simulink model "OberverForPMSM"  (R2018b)
settings: Solver=FixedStepAuto  StartTime=0.0  StopTime=inf  FixedStep=Ts  MaxStep=Ts  RelTol=1e-3  EnableMultiTasking=on
PreLoadFcn:
  | Ts=1e-6;
  | deci=20;
InitFcn:
  | Ts=5e-6;
  | deci=20;
undefined symbols (not defined in the file or in its folder): DiscIntNeverNeededParam, level
libraries: powerlib_extras x37, powerlib x18, powerlib_meascontrol x8, simulink x5, simulink_extras x4
(part 2 of 2)

== system OberverForPMSM/PMSG Wind Turbine/Control/Speed Control ==
  note: Speed Regulator
      | (Torque control)
  wr : Inport
  Enable : EnablePort
  0-inf1 : Saturate  UpperLimit=1.2  LowerLimit=0.7
  Divide2 : Product  Inputs=*/  SampleTime=Ts
  Gain1 : Gain  Gain=1/1.1^3  SampleTime=Ts
  Gain2 : Gain  Gain=-1  SampleTime=Ts
  Pmax : Constant
  Saturation1 : Saturate  UpperLimit=1  LowerLimit=0
  Saturation2 : Saturate  UpperLimit=1.5  LowerLimit=0
  Switch1 : Switch  Threshold=1.1
  Tracking Curve1 : Fcn  Expr=u(1)^3
  Tem_cmd : Outport
  wires:
  wr/1 -> 0-inf1/1, Divide2/2
  Pmax/1 -> Switch1/1
  0-inf1/1 -> Switch1/2, Tracking Curve1/1
  Switch1/1 -> Saturation1/1
  Divide2/1 -> Saturation2/1
  Saturation1/1 -> Divide2/1
  Tracking Curve1/1 -> Gain1/1
  Gain1/1 -> Switch1/3
  Saturation2/1 -> Gain2/1
  Gain2/1 -> Tem_cmd/1

== system OberverForPMSM/PMSG Wind Turbine/SMO_my/LL_To_Ph ==
  LL : Inport
  Selector : Selector  InputPortWidth=3  IndexOptions=Index vector (dialog)  Indices=[3 1 2]  OutputSizes=1
  Sum7 : Sum  Inputs=|+-
  constant : Gain  Gain=1/3
  Ph : Outport
  wires:
  LL/1 -> Sum7/1, Selector/1
  Selector/1 -> Sum7/2
  constant/1 -> Ph/1
  Sum7/1 -> constant/1

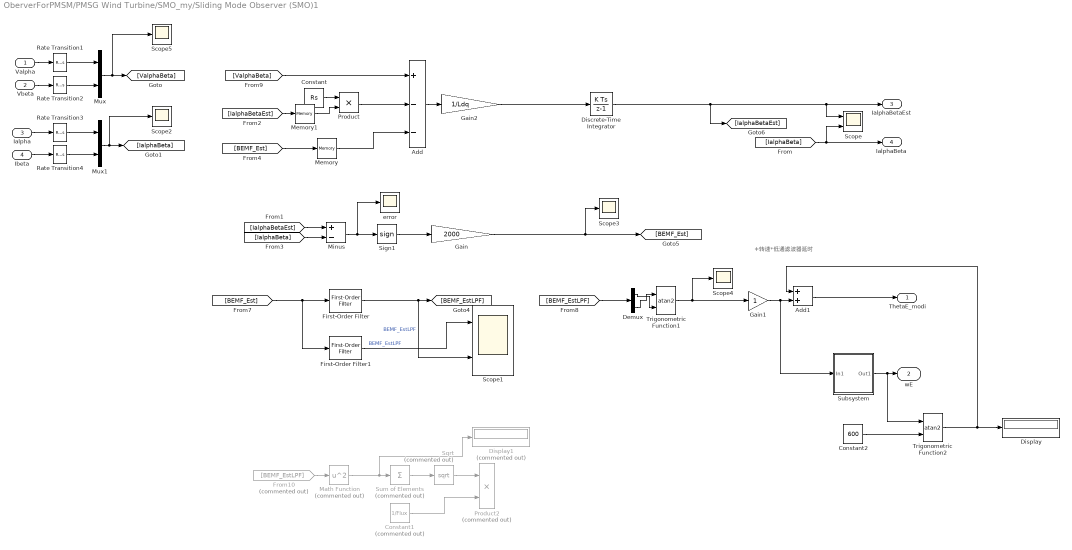
== system OberverForPMSM/PMSG Wind Turbine/SMO_my/Sliding Mode Observer (SMO)1 ==
  note: +转速*低通滤波器延时
  Valpha : Inport
  Vbeta : Inport  Port=2
  Ialpha : Inport  Port=3
  Ibeta : Inport  Port=4
  Add : Sum  Inputs=+--
  Add1 : Sum
  Constant : Constant  Value=Rs
  Constant1 : Constant  Commented=on  Value=1/Flux
  Constant2 : Constant  Value=600
  Demux : Demux  Outputs=2
  Discrete-Time Integrator : DiscreteIntegrator  SampleTime=-1  ICPrevOutput=DiscIntNeverNeededParam  ICPrevScaledInput=DiscIntNeverNeededParam
  Display : Display
  Display1 : Display  Commented=on
  First-Order Filter : powerlib_meascontrol/Filters/First-Order Filter  FilterType=Lowpass  Tc=1/600  Ts=Tctl  Initialize=on  Vac_Init=[0, 0, 60]  Vdc_Init=0  PlotResponse=off  FreqRange="[0,  200,  1]"
      settings: SourceProductName=Simscape Power Systems
  First-Order Filter1 : powerlib_meascontrol/Filters/First-Order Filter  FilterType=Lowpass  Tc=1/5000  Ts=Tctl  Initialize=on  Vac_Init=[0, 0, 60]  Vdc_Init=0  PlotResponse=off  FreqRange="[0,  200,  1]"
      settings: SourceProductName=Simscape Power Systems
  From10 : From  Commented=on  GotoTag=BEMF_EstLPF
  Gain : Gain  Gain=2000
  Gain1 : Gain
  Gain2 : Gain  Gain=1/Ldq
  Math Function : Math  Commented=on  Operator=square  SaturateOnIntegerOverflow=on
  Memory : Memory  InheritSampleTime=on
  Memory1 : Memory  InheritSampleTime=on
  Minus : Sum  Inputs=+-
  Mux : Mux  Inputs=2
  Mux1 : Mux  Inputs=2
  Product : Product
  Product2 : Product  Commented=on
  Rate Transition{1..4} (4 alike) : RateTransition  OutPortSampleTime=Tctl
  Scope : Scope  NumInputPorts=2
  Scope1 : Scope  NumInputPorts=2
  Scope{2..5} (4 alike) : Scope
  Sign1 : Signum
  Sqrt : Sqrt  Commented=on  SaturateOnIntegerOverflow=on
  Subsystem : Subsystem
  Sum of Elements : Sum  Commented=on  Inputs=+
  Trigonometric Function1 : Trigonometry  Operator=atan2  ApproximationMethod=CORDIC
  Trigonometric Function2 : Trigonometry  Operator=atan2  ApproximationMethod=CORDIC
  error : Scope
  ThetaE_modi : Outport
  wE : Outport  Port=2
  IalphaBetaEst : Outport  Port=3
  IalphaBeta : Outport  Port=4
  wires:
  Ibeta/1 -> Rate Transition4/1
  Ialpha/1 -> Rate Transition3/1
  Vbeta/1 -> Rate Transition2/1
  Valpha/1 -> Rate Transition1/1
  Mux/1 -> Scope5/1, [ValphaBeta]
  Mux1/1 -> Scope2/1, [IalphaBeta]
  [IalphaBetaEst] -> Minus/1
  [IalphaBeta] -> Minus/2
  [ValphaBeta] -> Add/1
  Constant/1 -> Product/1
  [IalphaBetaEst] -> Memory1/1
  Product/1 -> Add/2
  [BEMF_Est] -> Memory/1
  Add/1 -> Gain2/1
  Memory1/1 -> Product/2
  Gain2/1 -> Discrete-Time Integrator/1
  [IalphaBeta] -> Scope/2, IalphaBeta/1
  Minus/1 -> error/1, Sign1/1
  Memory/1 -> Add/3
  Sign1/1 -> Gain/1
  Gain/1 -> Scope3/1, [BEMF_Est]
  Trigonometric Function1/1 -> Scope4/1, Gain1/1
  Sum of Elements/1 -> Sqrt/1
  Math Function/1 -> Display1/1, Sum of Elements/1
  Sqrt/1 -> Product2/1
  Constant1/1 -> Product2/2
  From10/1 -> Math Function/1
  [BEMF_EstLPF] -> Demux/1
  Rate Transition1/1 -> Mux/1
  Rate Transition2/1 -> Mux/2
  Rate Transition3/1 -> Mux1/1
  Rate Transition4/1 -> Mux1/2
  [BEMF_Est] -> First-Order Filter1/1, First-Order Filter/1
  Discrete-Time Integrator/1 -> [IalphaBetaEst], Scope/1, IalphaBetaEst/1
  First-Order Filter/1 -> Scope1/2, [BEMF_EstLPF]  "BEMF_EstLPF"
  First-Order Filter1/1 -> Scope1/1  "BEMF_EstLPF"
  Subsystem/1(Out1) -> Trigonometric Function2/1, wE/1
  Demux/1 -> Trigonometric Function1/2
  Demux/2 -> Trigonometric Function1/1
  Gain1/1 -> Subsystem/1(In1), Add1/2
  Add1/1 -> ThetaE_modi/1
  Trigonometric Function2/1 -> Add1/1, Display/1
  Constant2/1 -> Trigonometric Function2/2

== system OberverForPMSM/PMSG Wind Turbine/SMO_my/mod 2 ==
  In1 : Inport
  Constant : Constant  Value=2*pi
  Math Function : Math  Operator=mod  SaturateOnIntegerOverflow=on
  Out1 : Outport
  wires:
  In1/1 -> Math Function/1
  Constant/1 -> Math Function/2
  Math Function/1 -> Out1/1

== system OberverForPMSM/PMSG Wind Turbine/SMO_my/mod 3 ==
  In1 : Inport
  Constant : Constant  Value=2*pi
  Math Function : Math  Operator=mod  SaturateOnIntegerOverflow=on
  Out1 : Outport
  wires:
  In1/1 -> Math Function/1
  Constant/1 -> Math Function/2
  Math Function/1 -> Out1/1

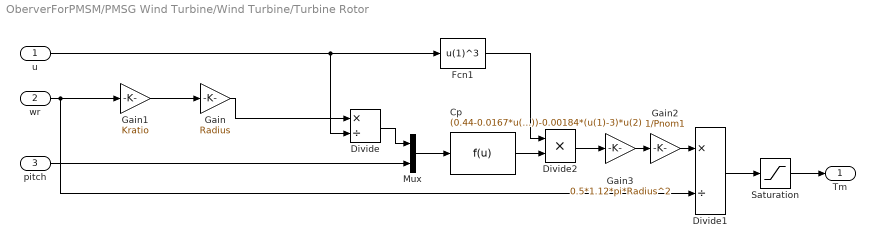
== system OberverForPMSM/PMSG Wind Turbine/Wind Turbine/Turbine Rotor ==
  u : Inport
  wr : Inport  Port=2
  pitch : Inport  Port=3
  Cp : Fcn  Expr=(0.44-0.0167*u(2))*sin(pi*(u(1)-3)/15-0.3*u(2))-0.00184*(u(1)-3)*u(2)  SampleTime=Ts
  Divide : Product  Inputs=*/  SampleTime=Ts
  Divide1 : Product  Inputs=*/  SampleTime=Ts
  Divide2 : Product  Inputs=**  SampleTime=Ts
  Fcn1 : Fcn  Expr=u(1)^3  SampleTime=Ts
  Gain : Gain  Gain=Radius  SampleTime=Ts
  Gain1 : Gain  Gain=Kratio  SampleTime=Ts
  Gain2 : Gain  Gain=1/Pnom1  SampleTime=Ts
  Gain3 : Gain  Gain=0.5*1.12*pi*Radius^2  SampleTime=Ts
  Mux : Mux  Inputs=2
  Saturation : Saturate  UpperLimit=2  LowerLimit=1e-2
  Tm : Outport
  wires:
  Gain/1 -> Divide/1
  u/1 -> Divide/2, Fcn1/1
  Divide/1 -> Mux/1
  Mux/1 -> Cp/1
  wr/1 -> Gain1/1, Divide1/2
  Gain1/1 -> Gain/1
  Gain2/1 -> Divide1/1
  Gain3/1 -> Gain2/1
  Divide2/1 -> Gain3/1
  Cp/1 -> Divide2/2
  Fcn1/1 -> Divide2/1
  pitch/1 -> Mux/2
  Divide1/1 -> Saturation/1
  Saturation/1 -> Tm/1

== system OberverForPMSM/PMSG Wind Turbine/Wind Turbine/pitch angle controller ==
  wg : Inport
  Ref : Inport  Port=2
  "0-pitch_max " : Saturate  UpperLimit=27  LowerLimit=0  SampleTime=Ts
  Discrete PID Controller : simulink/Continuous/PID Controller  Controller=P  Form=Parallel  TimeDomain=Discrete-time  SampleTime=Ts  IntegratorMethod=Forward Euler  FilterMethod=Forward Euler  ControllerParametersSource=internal  P=200  I=0  D=0  UseFilter=on  N=100  TunerSelectOption=Transfer Function Based (PID Tuner App)  ZeroCross=off  InitialConditionSource=internal  InitialConditionForIntegrator=0  InitialConditionForFilter=0  DifferentiatorICPrevScaledInput=0  ExternalReset=none  TrackingMode=off  Kt=1  LimitOutput=on  UpperSaturationLimit=27  LowerSaturationLimit=0  LinearizeAsGain=off  AntiWindupMode=clamping  Kb=1  POutMin=[]  POutMax=[]  IOutMin=[]  IOutMax=[]  DOutMin=[]  DOutMax=[]  NOutMin=[]  NOutMax=[]  SumOutMin=[]  SumOutMax=[]  SaturationOutMin=[]  SaturationOutMax=[]  PParamMin=[]  PParamMax=[]  IParamMin=[]  IParamMax=[]  DParamMin=[]  DParamMax=[]  NParamMin=[]  NParamMax=[]  KbParamMin=[]  KbParamMax=[]  KtParamMin=[]  KtParamMax=[]  KbOutMin=[]  KbOutMax=[]  KtOutMin=[]  KtOutMax=[]  IntegratorOutMin=[]  IntegratorOutMax=[]  FilterOutMin=[]  FilterOutMax=[]  SumI1OutMin=[]  SumI1OutMax=[]  SumI2OutMin=[]  SumI2OutMax=[]  SumI3OutMin=[]  SumI3OutMax=[]  SumI4OutMin=[]  SumI4OutMax=[]  SumDOutMin=[]  SumDOutMax=[]  DifferentiatorOutMin=[]  DifferentiatorOutMax=[]  FilterDiffOutCoefMin=[]  FilterDiffOutCoefMax=[]  ReciprocalOutMin=[]  ReciprocalOutMax=[]  SumDenOutMin=[]  SumDenOutMax=[]  SumNumOutMin=[]  SumNumOutMax=[]  DivideOutMin=[]  DivideOutMax=[]  IntegratorContinuousStateAttributes=''  IntegratorStateMustResolveToSignalObject=off  IntegratorRTWStateStorageClass=Auto  FilterContinuousStateAttributes=''  FilterStateMustResolveToSignalObject=off  FilterRTWStateStorageClass=Auto  ParallelPVariant=InternalParameters  IdealPVariant=Disabled  IVariant=Disabled  DVariant=Disabled  IntegratorVariant=Disabled  SatVariant=Enabled  AWVariant=Disabled  PCopyVariant=Disabled  TRVariant=Disabled  FdbkBlocksVariant=Forward  IdealPFdbkVariant=Disabled  SatFdbkVariant=Disabled  DerivativeFilterVariant=Disabled  NVariant=Disabled  NCopyVariant=Disabled_SignalSpec  FilterICVariant=Disabled  IntegratorICVariant=Disabled  ExternalResetVariant=Disabled  TRSumVariant=Passthrough  SumFdbkVariant=Disabled  SumVariant=Passthrough_P
  Rate Limiter : RateLimiter  RisingSlewLimit=10  FallingSlewLimit=-10
  Sum3 : Sum  Inputs=|+-  SampleTime=Ts
  t=Pitch_time_constant1 : powerlib_extras/Discrete  Control Blocks/Discrete 1st-Order Filter  FilterType=Lowpass  Tc=0.02  Ts=Ts  Initialize=on  Vac_Init=[0.8 -25 60]*0  Vdc_Init=0  PlotResponse=off  param1=[1 500 0.1]
  pitch : Outport
  wires:
  Sum3/1 -> Discrete PID Controller/1
  wg/1 -> Sum3/1
  Ref/1 -> Sum3/2
  Rate Limiter/1 -> "0-pitch_max "/1
  "0-pitch_max "/1 -> t=Pitch_time_constant1/1
  t=Pitch_time_constant1/1 -> pitch/1
  Discrete PID Controller/1 -> Rate Limiter/1

== system OberverForPMSM/PMSG Wind Turbine/ZhiQianChen/LL_To_Ph ==
  LL : Inport
  Selector : Selector  InputPortWidth=3  IndexOptions=Index vector (dialog)  Indices=[3 1 2]  OutputSizes=1
  Sum7 : Sum  Inputs=|+-
  constant : Gain  Gain=1/3
  Ph : Outport
  wires:
  Sum7/1 -> constant/1
  constant/1 -> Ph/1
  Selector/1 -> Sum7/2
  LL/1 -> Selector/1, Sum7/1

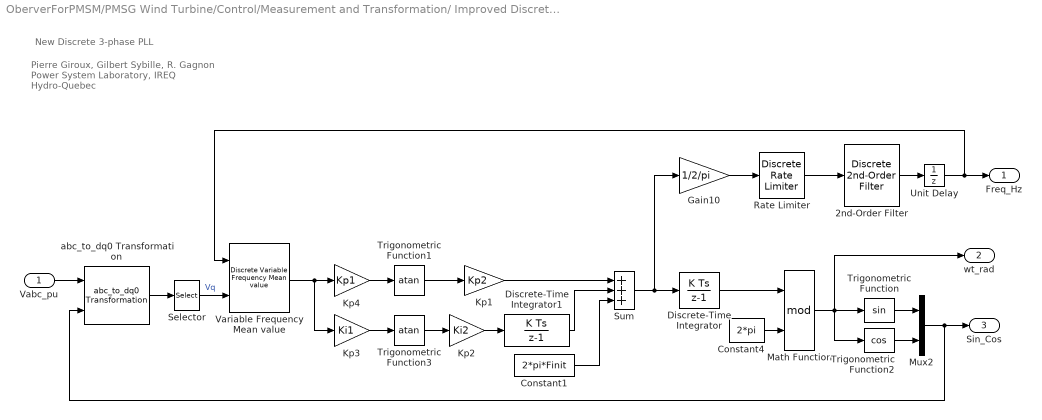
== system OberverForPMSM/PMSG Wind Turbine/Control/Measurement and Transformation/ Improved Discrete 3-phase PLL ==
  note: New Discrete 3-phase PLL
  note: Pierre Giroux, Gilbert Sybille, R. Gagnon
      | Power System Laboratory, IREQ
      | Hydro-Quebec
  Vabc_pu : Inport  PortDimensions=3
  2nd-Order Filter : powerlib_extras/Discrete  Control Blocks/Discrete  2nd-Order Filter  FilterType=Lowpass  Fo=25  Zeta=0.707  Ts=Ts  Initialize=on  Vac_Init=[0 0 Finit]  Vdc_Init=Finit  PlotResponse=off  param1=[1 500 0.1]
  Constant1 : Constant  Value=2*pi*Finit
  Constant4 : Constant  Value=2*pi
  Discrete-Time Integrator : DiscreteIntegrator  SampleTime=Ts  ICPrevOutput=DiscIntNeverNeededParam  ICPrevScaledInput=DiscIntNeverNeededParam
  Discrete-Time Integrator1 : DiscreteIntegrator  gainval=1  SampleTime=Ts  LimitOutput=on  UpperSaturationLimit=2*pi*5  LowerSaturationLimit=-2*pi*5  ICPrevOutput=DiscIntNeverNeededParam  ICPrevScaledInput=DiscIntNeverNeededParam
  Gain10 : Gain  Gain=1/2/pi  SaturateOnIntegerOverflow=on  OutDataTypeStr=Inherit: Same as input  ParamDataTypeStr=Inherit: Same as input
  Kp1 : Gain  Gain=Kp2  SaturateOnIntegerOverflow=on  OutDataTypeStr=Inherit: Same as input  ParamDataTypeStr=Inherit: Same as input
  Kp2 : Gain  Gain=Ki2  SaturateOnIntegerOverflow=on  OutDataTypeStr=Inherit: Same as input  ParamDataTypeStr=Inherit: Same as input
  Kp3 : Gain  Gain=Ki1  SaturateOnIntegerOverflow=on  OutDataTypeStr=Inherit: Same as input  ParamDataTypeStr=Inherit: Same as input
  Kp4 : Gain  Gain=Kp1  SaturateOnIntegerOverflow=on  OutDataTypeStr=Inherit: Same as input  ParamDataTypeStr=Inherit: Same as input
  Math Function : Math  Operator=mod  SaturateOnIntegerOverflow=on
  Mux2 : Mux  Inputs=2
  Rate Limiter : powerlib_extras/Discrete  Control Blocks/Discrete Rate Limiter  R=12  F=-12  Vinit=Finit  Ts=Ts
  Selector : Selector  InputPortWidth=3  IndexOptions=Index vector (dialog)  Indices=2  OutputSizes=1
  Sum : Sum  Inputs=+++
  Trigonometric Function : Trigonometry
  Trigonometric Function1 : Trigonometry  Operator=atan
  Trigonometric Function2 : Trigonometry  Operator=cos
  Trigonometric Function3 : Trigonometry  Operator=atan
  Unit Delay : UnitDelay  InitialCondition=Finit  SampleTime=Ts
  Variable Frequency Mean value : powerlib_extras/Discrete Measurements/Discrete Variable Frequency Mean value  Finit=Finit  Fmin=Fmin  Vinit=0  Ts=Ts
  abc_to_dq0 Transformation : powerlib_extras/Measurements/abc_to_dq0 Transformation
  Freq_Hz : Outport
  wt_rad : Outport  Port=2
  Sin_Cos : Outport  Port=3
  wires:
  Vabc_pu/1 -> abc_to_dq0 Transformation/1
  abc_to_dq0 Transformation/1 -> Selector/1
  Constant4/1 -> Math Function/2
  Math Function/1 -> Trigonometric Function/1, Trigonometric Function2/1, wt_rad/1
  Trigonometric Function/1 -> Mux2/1
  Trigonometric Function2/1 -> Mux2/2
  Mux2/1 -> Sin_Cos/1, abc_to_dq0 Transformation/2
  Gain10/1 -> Rate Limiter/1
  Rate Limiter/1 -> 2nd-Order Filter/1
  2nd-Order Filter/1 -> Unit Delay/1
  Selector/1 -> Variable Frequency Mean value/2  "Vq"
  Kp4/1 -> Trigonometric Function1/1
  Trigonometric Function1/1 -> Kp1/1
  Constant1/1 -> Sum/3
  Variable Frequency Mean value/1 -> Kp4/1, Kp3/1
  Kp3/1 -> Trigonometric Function3/1
  Trigonometric Function3/1 -> Kp2/1
  Kp2/1 -> Discrete-Time Integrator1/1
  Sum/1 -> Discrete-Time Integrator/1, Gain10/1
  Unit Delay/1 -> Freq_Hz/1, Variable Frequency Mean value/1
  Discrete-Time Integrator/1 -> Math Function/1
  Kp1/1 -> Sum/1
  Discrete-Time Integrator1/1 -> Sum/2

== system OberverForPMSM/PMSG Wind Turbine/Control/Measurement and Transformation/ABC to dq conversion  ==
  abc : Inport
  Teta : Inport  Port=2
  Fcn : Fcn  Expr=sin(u)
  Fcn1 : Fcn  Expr=cos(u)
  Gain : Gain  Gain=2/3  SaturateOnIntegerOverflow=on  OutDataTypeStr=Inherit: Same as input  ParamDataTypeStr=Inherit: Same as input
  Gain1 : Gain  Gain=2/3  SaturateOnIntegerOverflow=on  OutDataTypeStr=Inherit: Same as input  ParamDataTypeStr=Inherit: Same as input
  Mux : Mux  Inputs=[1 1 3]
  id : Fcn  Expr=u[1]*u[3]+(1.7320508*u[2]-u[1])*u[4]*0.5+(-u[1]-1.7320508*u[2])*u[5]*0.5
  iq : Fcn  Expr=-u[2]*u[3]+(u[2]+1.7320508*u[1])*u[4]*0.5+(u[2]-1.7320508*u[1])*u[5]*0.5
  d : Outport  InitialOutput=0
  q : Outport  Port=2  InitialOutput=0
  wires:
  Fcn/1 -> Mux/2
  Fcn1/1 -> Mux/1
  Teta/1 -> Fcn1/1, Fcn/1
  Mux/1 -> iq/1, id/1
  abc/1 -> Mux/3
  iq/1 -> Gain1/1
  id/1 -> Gain/1
  Gain/1 -> d/1
  Gain1/1 -> q/1

== system OberverForPMSM/PMSG Wind Turbine/Control/Measurement and Transformation/ABC to dq conversion ==
  abc : Inport
  Teta : Inport  Port=2
  Fcn : Fcn  Expr=sin(u)
  Fcn1 : Fcn  Expr=cos(u)
  Gain : Gain  Gain=2/3  SaturateOnIntegerOverflow=on  OutDataTypeStr=Inherit: Same as input  ParamDataTypeStr=Inherit: Same as input
  Gain1 : Gain  Gain=2/3  SaturateOnIntegerOverflow=on  OutDataTypeStr=Inherit: Same as input  ParamDataTypeStr=Inherit: Same as input
  Mux : Mux  Inputs=[1 1 3]
  id : Fcn  Expr=u[1]*u[3]+(1.7320508*u[2]-u[1])*u[4]*0.5+(-u[1]-1.7320508*u[2])*u[5]*0.5
  iq : Fcn  Expr=-u[2]*u[3]+(u[2]+1.7320508*u[1])*u[4]*0.5+(u[2]-1.7320508*u[1])*u[5]*0.5
  d : Outport  InitialOutput=0
  q : Outport  Port=2  InitialOutput=0
  wires:
  Fcn/1 -> Mux/2
  Fcn1/1 -> Mux/1
  Teta/1 -> Fcn1/1, Fcn/1
  Mux/1 -> iq/1, id/1
  abc/1 -> Mux/3
  iq/1 -> Gain1/1
  id/1 -> Gain/1
  Gain/1 -> d/1
  Gain1/1 -> q/1

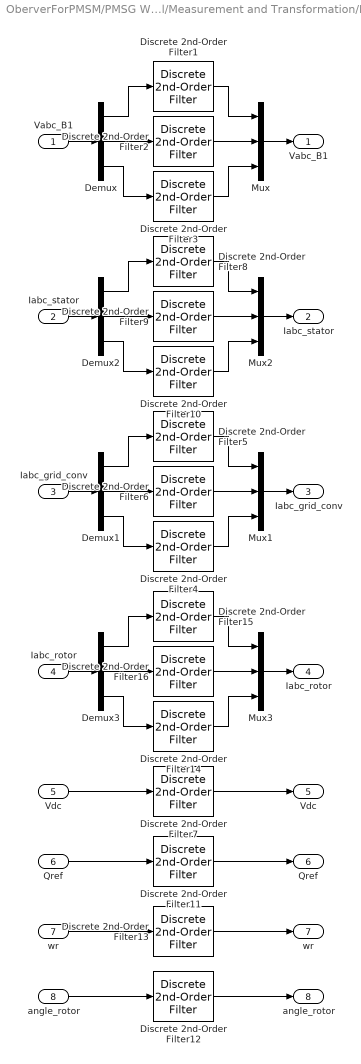
== system OberverForPMSM/PMSG Wind Turbine/Control/Measurement and Transformation/Filter ==
  Vabc_B1 : Inport
  Iabc_stator : Inport  Port=2
  Iabc_grid_conv : Inport  Port=3
  Iabc_rotor : Inport  Port=4
  Vdc : Inport  Port=5
  Qref : Inport  Port=6
  wr : Inport  Port=7
  angle_rotor : Inport  Port=8
  Demux{,1..3} (4 alike) : Demux  Outputs=3
  Discrete 2nd-Order Filter{1..6,8..16} (15 alike) : powerlib_extras/Discrete  Control Blocks/Discrete  2nd-Order Filter  FilterType=Lowpass  Fo=Freq  Zeta=Zeta1  Ts=Ts  Initialize=off  Vac_Init=[0.8 -25 60]  Vdc_Init=-0.4  PlotResponse=off  param1=[1 500 1]
  Discrete 2nd-Order Filter7 : powerlib_extras/Discrete  Control Blocks/Discrete  2nd-Order Filter  FilterType=Lowpass  Fo=Freq  Zeta=Zeta1  Ts=Ts  Initialize=on  Vac_Init=[0.8 -25 60]*0  Vdc_Init=Vdc_nom  PlotResponse=off  param1=[1 500 1]
  Mux{,1..3} (4 alike) : Mux  Inputs=3
  "Vabc_B1 " : Outport
  "Iabc_stator " : Outport  Port=2
  "Iabc_grid_conv " : Outport  Port=3
  "Iabc_rotor " : Outport  Port=4
  "Vdc " : Outport  Port=5
  "Qref " : Outport  Port=6
  "wr " : Outport  Port=7
  "angle_rotor " : Outport  Port=8
  wires:
  Discrete 2nd-Order Filter12/1 -> "angle_rotor "/1
  angle_rotor/1 -> Discrete 2nd-Order Filter12/1
  Discrete 2nd-Order Filter11/1 -> "Qref "/1
  Qref/1 -> Discrete 2nd-Order Filter11/1
  Mux3/1 -> "Iabc_rotor "/1
  Iabc_rotor/1 -> Demux3/1
  Discrete 2nd-Order Filter14/1 -> Mux3/3
  Discrete 2nd-Order Filter16/1 -> Mux3/2
  Discrete 2nd-Order Filter15/1 -> Mux3/1
  Demux3/3 -> Discrete 2nd-Order Filter14/1
  Demux3/2 -> Discrete 2nd-Order Filter16/1
  Demux3/1 -> Discrete 2nd-Order Filter15/1
  Discrete 2nd-Order Filter13/1 -> "wr "/1
  wr/1 -> Discrete 2nd-Order Filter13/1
  Mux2/1 -> "Iabc_stator "/1
  Iabc_stator/1 -> Demux2/1
  Discrete 2nd-Order Filter10/1 -> Mux2/3
  Discrete 2nd-Order Filter9/1 -> Mux2/2
  Discrete 2nd-Order Filter8/1 -> Mux2/1
  Demux2/3 -> Discrete 2nd-Order Filter10/1
  Demux2/2 -> Discrete 2nd-Order Filter9/1
  Demux2/1 -> Discrete 2nd-Order Filter8/1
  Discrete 2nd-Order Filter7/1 -> "Vdc "/1
  Vdc/1 -> Discrete 2nd-Order Filter7/1
  Mux1/1 -> "Iabc_grid_conv "/1
  Iabc_grid_conv/1 -> Demux1/1
  Discrete 2nd-Order Filter4/1 -> Mux1/3
  Discrete 2nd-Order Filter6/1 -> Mux1/2
  Discrete 2nd-Order Filter5/1 -> Mux1/1
  Demux1/3 -> Discrete 2nd-Order Filter4/1
  Demux1/2 -> Discrete 2nd-Order Filter6/1
  Demux1/1 -> Discrete 2nd-Order Filter5/1
  Mux/1 -> "Vabc_B1 "/1
  Vabc_B1/1 -> Demux/1
  Discrete 2nd-Order Filter3/1 -> Mux/3
  Discrete 2nd-Order Filter2/1 -> Mux/2
  Discrete 2nd-Order Filter1/1 -> Mux/1
  Demux/3 -> Discrete 2nd-Order Filter3/1
  Demux/2 -> Discrete 2nd-Order Filter2/1
  Demux/1 -> Discrete 2nd-Order Filter1/1

== system OberverForPMSM/PMSG Wind Turbine/Control/Rotor-side Controls/dq to ABC conversion  ==
  dq : Inport
  Teta : Inport  Port=2
  Fcn : Fcn  Expr=sin(u)
  Fcn1 : Fcn  Expr=cos(u)
  Mux : Mux  Inputs=[1 1 2]
  Mux1 : Mux  Inputs=3
  a : Fcn  Expr=u(1)*u(3)-u(2)*u(4)
  b : Fcn  Expr=(u(1)*(-0.5)+u(2)*(0.8660254))*u(3)-(u(2)*(-0.5)-u(1)*(0.8660254))*u(4)
  c : Fcn  Expr=(u(1)*(-0.5)-u(2)*(0.8660254))*u(3)-(u(2)*(-0.5)+u(1)*(0.8660254))*u(4)
  ABC : Outport
  wires:
  Fcn/1 -> Mux/2
  Fcn1/1 -> Mux/1
  Teta/1 -> Fcn1/1, Fcn/1
  Mux/1 -> a/1, b/1, c/1
  dq/1 -> Mux/3
  b/1 -> Mux1/2
  a/1 -> Mux1/1
  Mux1/1 -> ABC/1
  c/1 -> Mux1/3

== system OberverForPMSM/PMSG Wind Turbine/Control/Rotor-side Controls/dq to ABC conversion 1 ==
  dq : Inport
  Teta : Inport  Port=2
  Fcn : Fcn  Expr=sin(u)
  Fcn1 : Fcn  Expr=cos(u)
  Mux : Mux  Inputs=[1 1 2]
  Mux1 : Mux  Inputs=3
  a : Fcn  Expr=u(1)*u(3)-u(2)*u(4)
  b : Fcn  Expr=(u(1)*(-0.5)+u(2)*(0.8660254))*u(3)-(u(2)*(-0.5)-u(1)*(0.8660254))*u(4)
  c : Fcn  Expr=(u(1)*(-0.5)-u(2)*(0.8660254))*u(3)-(u(2)*(-0.5)+u(1)*(0.8660254))*u(4)
  ABC : Outport
  wires:
  Fcn/1 -> Mux/2
  Fcn1/1 -> Mux/1
  Teta/1 -> Fcn1/1, Fcn/1
  Mux/1 -> a/1, b/1, c/1
  dq/1 -> Mux/3
  b/1 -> Mux1/2
  a/1 -> Mux1/1
  Mux1/1 -> ABC/1
  c/1 -> Mux1/3

== system OberverForPMSM/PMSG Wind Turbine/SMO_my/Sliding Mode Observer (SMO)1/Subsystem ==
  note: Dtheta/Dt
      | =speed
  note: 角度增量
  In1 : Inport
  Discrete Derivative1 : simulink/Discrete/Discrete Derivative  gainval=1.0  ICPrevScaledInput=0.0  OutMin=[]  OutMax=[]  OutDataType=fixdt(1, 16)  OutScaling=2^-10  DoSatur=off
  First-Order Filter1 : powerlib_meascontrol/Filters/First-Order Filter  FilterType=Lowpass  Tc=1/50  Ts=Tctl  Initialize=on  Vac_Init=[0, 0, 60]  Vdc_Init=0  PlotResponse=off  FreqRange="[0,  200,  1]"
      settings: SourceProductName=Simscape Power Systems
  Gain : Gain  Gain=1/Tctl
  MATLAB Function : MATLAB Function  TreatAsAtomicUnit=on
  Memory1 : Memory  InheritSampleTime=on
  Memory2 : Memory  InheritSampleTime=on
  Minus : Sum  Inputs=+-
  Scope : Scope  NumInputPorts=2
  Out1 : Outport
  wires:
  In1/1 -> Memory1/1, Minus/1
  Memory1/1 -> Minus/2
  MATLAB Function/1(dThetaOut) -> Memory2/1, Scope/2, Gain/1
  Minus/1 -> Scope/1, MATLAB Function/1(dTheta)
  Memory2/1 -> MATLAB Function/2(dThetaLast)
  First-Order Filter1/1 -> Out1/1  "BEMF_EstLPF"
  Gain/1 -> First-Order Filter1/1

== matlab function OberverForPMSM/PMSG Wind Turbine/ZhiQianChen/MATLAB Function ==
  data: g1 input; delta_xi output; g2 input; omega_e input; R_s input; Ld input; Lq input; xi input; u_alphabeta input; i_alphabeta input; EMF output
function [delta_xi,EMF]  = zhiqianChen(g1,g2,omega_e,R_s,Ld,Lq,xi,u_alphabeta,i_alphabeta)
    delta_xi = [0;0];
    EMF = [0;0];
    %pξ=    A_0 ξ   +   A_1 i   +   A_2 u
    %A_0=   G/L_d+ω_re  J 
    %A_1=   ω_re  JG+G(R_s-∆Lω_re J+G)/L_d
    %A_2=   - G/L_d
    G = [g1 -g2;
        g2 g1];
    I = [1 0;
        0 1];
    J = [0 -1;
        1 0];
    
    A_0 = G/Ld + omega_e*J;
    A_1 = omega_e*J*G + G*(R_s-(Ld-Lq)*omega_e*J +G)/Ld;
    A_2 = -G/Ld;
    delta_xi = A_0*xi + A_1*i_alphabeta + A_2*u_alphabeta;
    EMF = xi + G*i_alphabeta;

end

== matlab function OberverForPMSM/PMSG Wind Turbine/SMO_my/Sliding Mode Observer (SMO)1/Subsystem/MATLAB Function ==
  data: dTheta input; dThetaOut output; dThetaLast input
function dThetaOut = fcn(dTheta,dThetaLast)

dThetaOut = 0;

if abs(dTheta - dThetaLast) < 0.1
    dThetaOut =  dTheta;
elseif abs(dTheta - dThetaLast + 2*pi) < 0.1
    dThetaOut =  dTheta + 2*pi;
elseif abs(dTheta - dThetaLast - 2*pi) < 0.1
    dThetaOut =  dTheta - 2*pi;
else
    dThetaOut =  dThetaLast;
end

end
